simulink model "Simulation_DCModel"  (R2021a)
settings: Solver=ode5  StartTime=ti  StopTime=tf  FixedStep=Ts/40  RelTol=1e-3
undefined symbols (not defined in the file): A_real, B_real, Cx_real, Dx_real, f, IC, Noise, torque, u0, umax
libraries: simulink x1
settings Model: Creator=perruquetti  LastModifiedBy=perruquetti
settings SolverCC: AlgebraicLoopSolver=TrustRegion
settings DataIOCC: ReturnWorkspaceOutputs=off
settings DebuggingCC: SFMachineParentedDataDiag=warning  ArithmeticOperatorsInVariantConditions=warning
settings SFSimCC: SimUseLocalCustomCode=off  CustomCodeUndefinedFunction=UseInterfaceOnly
settings RTWCC: RTWUseLocalCustomCode=off

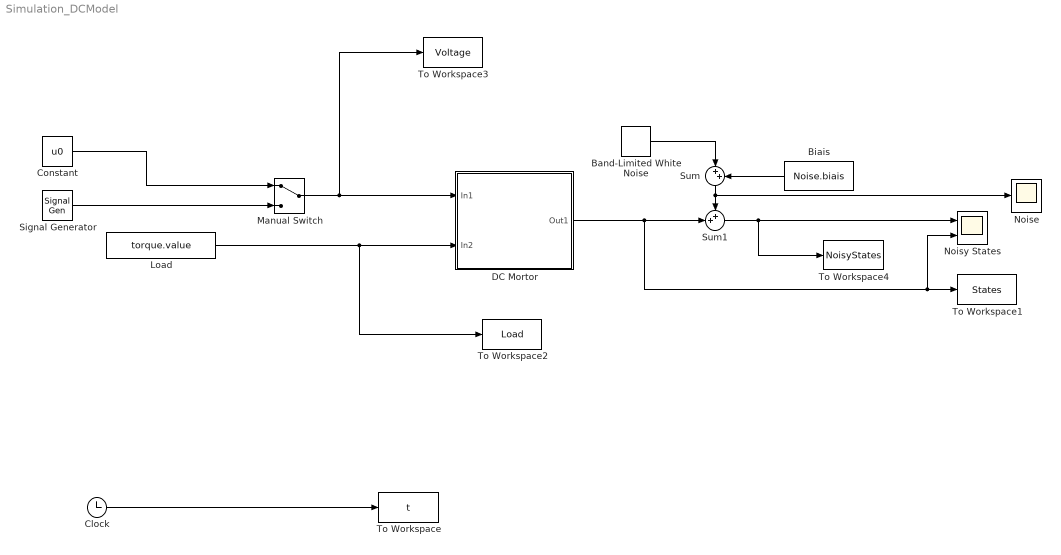
== system Simulation_DCModel ==
  Band-Limited White Noise : simulink/Sources/Band-Limited White Noise  Cov=Noise.power  Ts=Noise.sampling  seed=Noise.seed
  Biais : Constant  Value=Noise.biais
  Clock : Clock
  Constant : Constant  Value=u0
  DC Mortor : Subsystem
      mask Display: image('motor2.png');
  Load : Constant  Value=torque.value
  Manual Switch : ManualSwitch
  Noise : Scope
  Noisy States : Scope  NumInputPorts=2
  Signal Generator : SignalGenerator  Amplitude=u0  Frequency=f  Units=rad/sec
  Sum : Sum  Inputs=|++
  Sum1 : Sum  Inputs=++|
  To Workspace : ToWorkspace  VariableName=t  SampleTime=-1
  To Workspace1 : ToWorkspace  VariableName=States  SampleTime=-1
  To Workspace2 : ToWorkspace  VariableName=Load  SampleTime=-1
  To Workspace3 : ToWorkspace  VariableName=Voltage  SampleTime=-1
  To Workspace4 : ToWorkspace  VariableName=NoisyStates  SampleTime=-1
  wires:
  Band-Limited White Noise/1 -> Sum/1
  Biais/1 -> Sum/2
  Sum/1 -> Noise/1, Sum1/1
  Sum1/1 -> To Workspace4/1, Noisy States/1
  Clock/1 -> To Workspace/1
  DC Mortor/1(Out1) -> Noisy States/2, To Workspace1/1, Sum1/2
  Load/1 -> To Workspace2/1, DC Mortor/2(In2)
  Constant/1 -> Manual Switch/1
  Signal Generator/1 -> Manual Switch/2
  Manual Switch/1 -> To Workspace3/1, DC Mortor/1(In1)

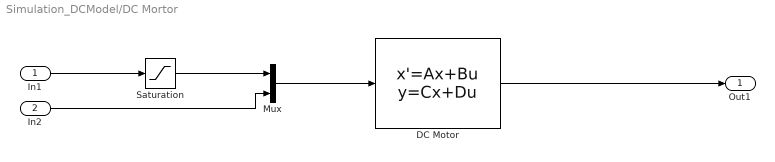
== system Simulation_DCModel/DC Mortor ==
  In1 : Inport
  In2 : Inport  Port=2
  DC Motor : StateSpace  A=A_real  B=B_real  C=Cx_real  D=Dx_real  InitialCondition=IC.state
  Mux : Mux  Inputs=2
  Saturation : Saturate  UpperLimit=umax  LowerLimit=-umax
  Out1 : Outport  VectorParamsAs1DForOutWhenUnconnected=off
  wires:
  DC Motor/1 -> Out1/1
  In1/1 -> Saturation/1
  Saturation/1 -> Mux/1
  Mux/1 -> DC Motor/1
  In2/1 -> Mux/2
